simulink model "hw3_b_ELS_model_extended_c05"  (R2024b)
settings: Solver=ode4  StartTime=0.0  StopTime=sim_time*10  FixedStep=sample_time  RelTol=1e-3
values from neighbouring files (symbols this model uses):
  a = -0.8    [hw3_a_rls_v2.m]    (also in hw3_b_rls_v2.m)
  b = 0.5    [hw3_a_rls_v2.m]    (also in hw3_b_rls_v2.m)
  c = -0.5    [hw3_a_rls_v2.m]    (also in hw3_b_rls_v2.m = 0)
  noise_mean = 0    [hw3_a_rls_v2.m]    (also in hw3_b_rls_v2.m)
  noise_seed = round(rand*1e5)    [hw3_a_rls_v2.m]    (also in hw3_b_rls_v2.m)
  noise_variance = 0.5    [hw3_a_rls_v2.m]    (also in hw3_b_rls_v2.m)
  sample_time = 1    [hw3_a_rls_v2.m]    (also in hw3_b_rls_v2.m)
libraries: simulink x1
settings Model: Creator=kemal  LastModifiedBy=kemal

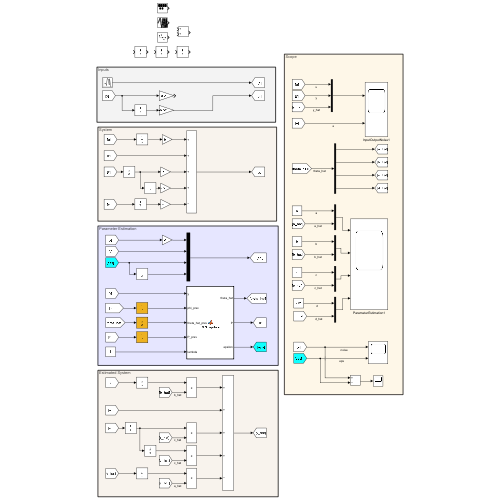
[thumbnail: Simulink's stored preview of the top-level diagram]
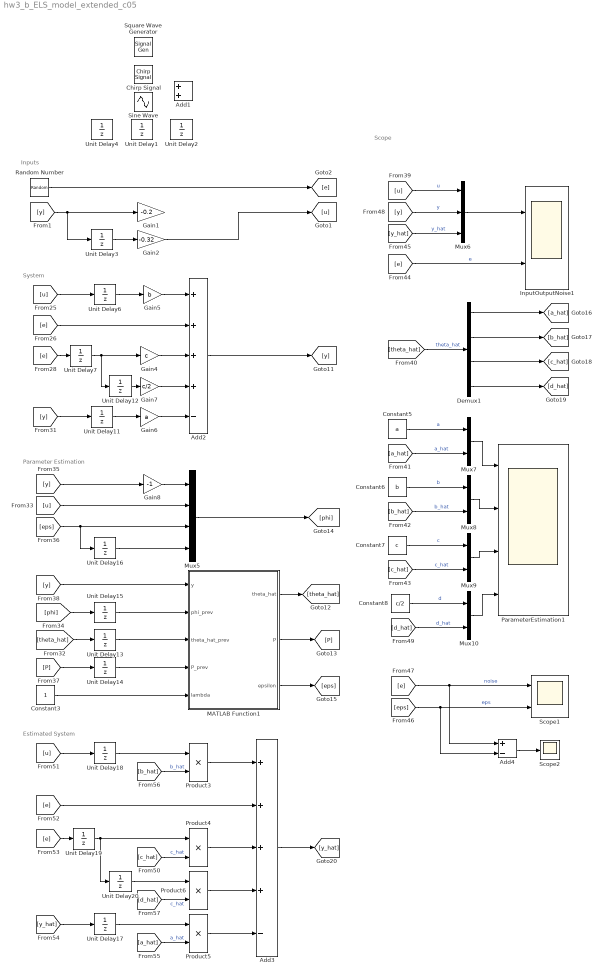
== system hw3_b_ELS_model_extended_c05 ==
  note: System
  note: Parameter Estimation
  note: Scope
  note: Estimated System
  note: Inputs
  Add1 : Sum
  Add2 : Sum  Inputs=++++-
  Add3 : Sum  Inputs=++++-
  Add4 : Sum  Inputs=+-
  Chirp Signal : simulink/Sources/Chirp Signal  f1=0.1  T=100  f2=1000
  Constant3 : Constant  SampleTime=-1
  Constant5 : Constant  Value=a  SampleTime=sample_time
  Constant6 : Constant  Value=b  SampleTime=sample_time
  Constant7 : Constant  Value=c  SampleTime=sample_time
  Constant8 : Constant  Value=c/2  SampleTime=sample_time
  Demux1 : Demux
  Gain1 : Gain  Gain=-0.2
  Gain2 : Gain  Gain=-0.32
  Gain4 : Gain  Gain=c
  Gain5 : Gain  Gain=b
  Gain6 : Gain  Gain=a
  Gain7 : Gain  Gain=c/2
  Gain8 : Gain  Gain=-1
  InputOutputNoise1 : Scope  NumInputPorts=2
  MATLAB Function1 : MATLAB Function  TreatAsAtomicUnit=on
  Mux{7..10} (4 alike) : Mux  Inputs=2
  Mux5 : Mux
  Mux6 : Mux  Inputs=3
  ParameterEstimation1 : Scope  NumInputPorts=4
  Product{3..6} (4 alike) : Product
  Random Number : RandomNumber  Mean=noise_mean  Variance=noise_variance  Seed=noise_seed  SampleTime=sample_time
  Scope1 : Scope  NumInputPorts=2
  Scope2 : Scope
  Sine Wave : Sin  Amplitude=5  Frequency=2*pi/10  SampleTime=0
  Square Wave Generator : SignalGenerator  WaveForm=square  Frequency=1/100
  Unit Delay{1..4,6..7,11..12,16..20} (13 alike) : UnitDelay  SampleTime=sample_time  HasFrameUpgradeWarning=on
  Unit Delay13 : UnitDelay  InitialCondition=zeros(4,1)  SampleTime=sample_time  HasFrameUpgradeWarning=on
  Unit Delay14 : UnitDelay  InitialCondition=eye(4)*100  SampleTime=sample_time  HasFrameUpgradeWarning=on
  Unit Delay15 : UnitDelay  InitialCondition=zeros(4,1)  SampleTime=sample_time  HasFrameUpgradeWarning=on
  wires:
  Add2/1 -> [y]
  Gain6/1 -> Add2/5
  Unit Delay11/1 -> Gain6/1
  [y] -> Unit Delay11/1
  Gain5/1 -> Add2/1
  [e] -> Add2/2
  Gain4/1 -> Add2/3
  Unit Delay6/1 -> Gain5/1
  Unit Delay7/1 -> Unit Delay12/1, Gain4/1
  [e] -> Unit Delay7/1
  [u] -> Unit Delay6/1
  Unit Delay12/1 -> Gain7/1
  Gain7/1 -> Add2/4
  MATLAB Function1/3(epsilon) -> [eps]
  [eps] -> Unit Delay16/1, Mux5/3
  Unit Delay15/1 -> MATLAB Function1/2(phi_prev)
  [u] -> Mux5/2
  [phi] -> Unit Delay15/1
  Mux5/1 -> [phi]
  Gain8/1 -> Mux5/1
  [y] -> Gain8/1
  [y] -> MATLAB Function1/1(y)
  Constant3/1 -> MATLAB Function1/5(lambda)
  Unit Delay14/1 -> MATLAB Function1/4(P_prev)
  [P] -> Unit Delay14/1
  Unit Delay13/1 -> MATLAB Function1/3(theta_hat_prev)
  [theta_hat] -> Unit Delay13/1
  MATLAB Function1/1(theta_hat) -> [theta_hat]
  MATLAB Function1/2(P) -> [P]
  Unit Delay16/1 -> Mux5/4
  [e] -> Add4/1, Scope1/1  "noise"
  [eps] -> Add4/2, Scope1/2  "eps"
  [c_hat] -> Mux9/2  "c_hat"
  Demux1/3 -> [c_hat]
  Mux9/1 -> ParameterEstimation1/3
  Constant7/1 -> Mux9/1  "c"
  [y_hat] -> Mux6/3  "y_hat"
  [b_hat] -> Mux8/2  "b_hat"
  [a_hat] -> Mux7/2  "a_hat"
  Constant6/1 -> Mux8/1  "b"
  Demux1/2 -> [b_hat]
  Demux1/1 -> [a_hat]
  Constant5/1 -> Mux7/1  "a"
  Mux8/1 -> ParameterEstimation1/2
  Mux7/1 -> ParameterEstimation1/1
  [theta_hat] -> Demux1/1  "theta_hat"
  Mux6/1 -> InputOutputNoise1/1
  [e] -> InputOutputNoise1/2  "e"
  [y] -> Mux6/2  "y"
  [u] -> Mux6/1  "u"
  Demux1/4 -> [d_hat]
  Constant8/1 -> Mux10/1  "d"
  [d_hat] -> Mux10/2  "d_hat"
  Mux10/1 -> ParameterEstimation1/4
  Add3/1 -> [y_hat]
  [y_hat] -> Unit Delay17/1
  Unit Delay18/1 -> Product3/1
  [e] -> Unit Delay19/1
  [u] -> Unit Delay18/1
  Product3/1 -> Add3/1
  Product4/1 -> Add3/3
  Unit Delay19/1 -> Unit Delay20/1, Product4/1
  [b_hat] -> Product3/2  "b_hat"
  [c_hat] -> Product4/2  "c_hat"
  [a_hat] -> Product5/2  "a_hat"
  Unit Delay17/1 -> Product5/1
  [e] -> Add3/2
  [d_hat] -> Product6/2  "c_hat"
  Unit Delay20/1 -> Product6/1
  Product6/1 -> Add3/4
  Product5/1 -> Add3/5
  Add4/1 -> Scope2/1
  Gain2/1 -> [u]
  Unit Delay3/1 -> Gain2/1
  Random Number/1 -> [e]
  [y] -> Gain1/1, Unit Delay3/1

== matlab function hw3_b_ELS_model_extended_c05/MATLAB Function1 ==
  data: y input; theta_hat output; phi_prev input; theta_hat_prev input; P_prev input; lambda input; P output; epsilon output
function [theta_hat, P, epsilon] = RLS_update(y, phi_prev, theta_hat_prev, P_prev, lambda)
    % Compute innovation
    epsilon = y - phi_prev' * theta_hat_prev;
     
    % Update covariance matrix
    P = (1/lambda) * (P_prev - (P_prev * (phi_prev * phi_prev') * P_prev) / ...
        (lambda + phi_prev' * P_prev * phi_prev));

    % Update parameter estimate
    theta_hat = theta_hat_prev + P * phi_prev * epsilon;
end
